simulink model "suspension2DOF"  (R2025b)
settings: Solver=ode5  StartTime=0.0  StopTime=10.0  FixedStep=0.001  RelTol=1e-3
InitFcn:
  | % 悬架参数
  | m_s = 350;
  | m_u = 45;
  | k_s = 20000;
  | c_s = 1100;
  | k_t = 200000;
undefined symbols (not defined in the file): road
settings Model: Creator=23649  LastModifiedBy=23649

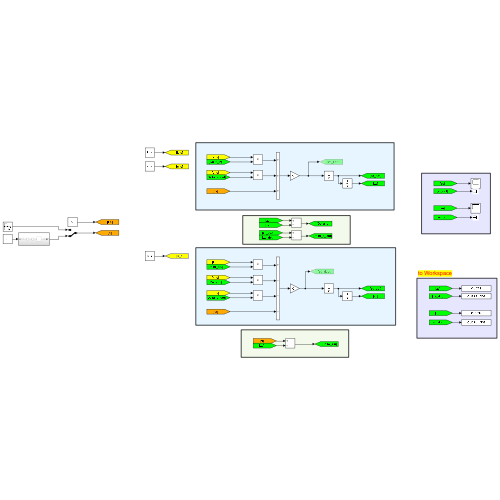
[thumbnail: Simulink's stored preview of the top-level diagram]
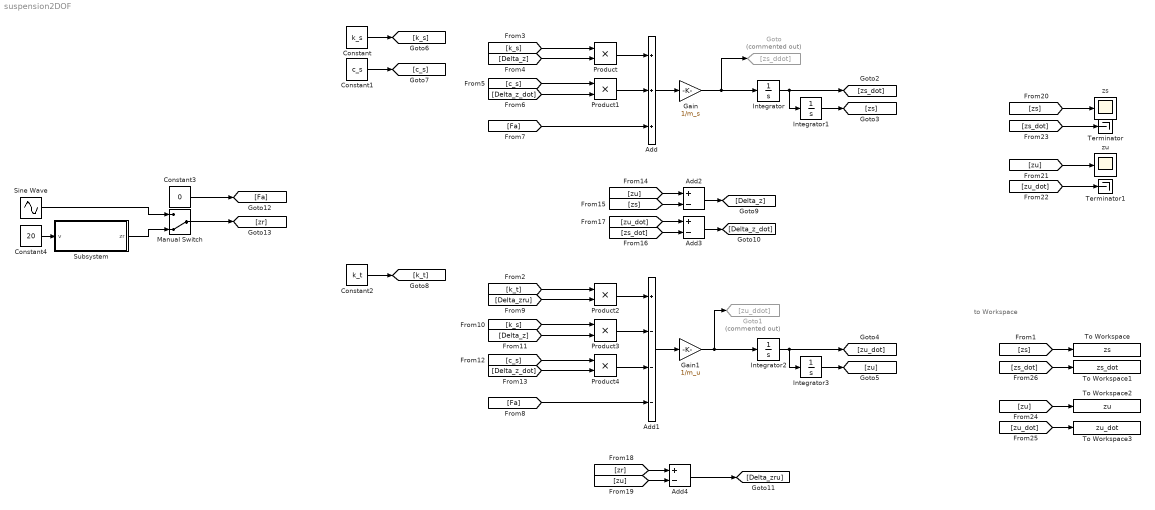
== system suspension2DOF ==
  note: to Workspace
  Add : Sum  Inputs=+++
  Add1 : Sum  Inputs=+---
  Add2 : Sum  Inputs=+-
  Add3 : Sum  Inputs=+-
  Add4 : Sum  Inputs=+-
  Constant : Constant  Value=k_s
  Constant1 : Constant  Value=c_s
  Constant2 : Constant  Value=k_t
  Constant3 : Constant  Value=0
  Constant4 : Constant  Value=20
  Gain : Gain  Gain=1/m_s
  Gain1 : Gain  Gain=1/m_u
  Goto : Goto  Commented=on  GotoTag=zs_ddot
  Goto1 : Goto  Commented=on  GotoTag=zu_ddot
  Integrator{,1..3} (4 alike) : Integrator
  Manual Switch : ManualSwitch  CurrentSetting=0
  Product{,1..4} (5 alike) : Product
  Sine Wave : Sin  Frequency=10  SampleTime=0
  Subsystem : Subsystem
  Terminator : Terminator
  Terminator1 : Terminator
  To Workspace : ToWorkspace  VariableName=zs  SampleTime=-1
  To Workspace1 : ToWorkspace  VariableName=zs_dot  SampleTime=-1
  To Workspace2 : ToWorkspace  VariableName=zu  SampleTime=-1
  To Workspace3 : ToWorkspace  VariableName=zu_dot  SampleTime=-1
  zs : Scope
      settings: ActiveDisplayYMinimum=-0.09781656463935004  ActiveDisplayYMaximum=0.084748231239210714
  zu : Scope
      settings: ActiveDisplayYMinimum=-0.097978742792255435  ActiveDisplayYMaximum=0.080113596148861266
  wires:
  Product/1 -> Add/1
  [Delta_z] -> Product/2
  [k_s] -> Product/1
  Product1/1 -> Add/2
  [Fa] -> Add/3
  [Delta_z_dot] -> Product1/2
  [c_s] -> Product1/1
  Add/1 -> Gain/1
  Gain/1 -> Goto/1, Integrator/1
  Integrator/1 -> [zs_dot], Integrator1/1
  Integrator1/1 -> [zs]
  Integrator3/1 -> [zu]
  Integrator2/1 -> Integrator3/1, [zu_dot]
  Gain1/1 -> Integrator2/1, Goto1/1
  Add1/1 -> Gain1/1
  [k_s] -> Product3/1
  [Delta_z] -> Product3/2
  Product3/1 -> Add1/2
  [k_t] -> Product2/1
  [Delta_zru] -> Product2/2
  Product2/1 -> Add1/1
  Constant/1 -> [k_s]
  Constant1/1 -> [c_s]
  Constant2/1 -> [k_t]
  [c_s] -> Product4/1
  [Delta_z_dot] -> Product4/2
  [Fa] -> Add1/4
  Product4/1 -> Add1/3
  [zu] -> Add2/1
  [zs] -> Add2/2
  Add2/1 -> [Delta_z]
  [zu_dot] -> Add3/1
  [zs_dot] -> Add3/2
  Add3/1 -> [Delta_z_dot]
  [zu] -> Add4/2
  [zr] -> Add4/1
  Add4/1 -> [Delta_zru]
  [zs] -> zs/1
  [zu] -> zu/1
  [zs_dot] -> Terminator/1
  [zu_dot] -> Terminator1/1
  Constant3/1 -> [Fa]
  Manual Switch/1 -> [zr]
  Constant4/1 -> Subsystem/1(v)
  Sine Wave/1 -> Manual Switch/1
  Subsystem/1(zr) -> Manual Switch/2
  [zs] -> To Workspace/1
  [zs_dot] -> To Workspace1/1
  [zu] -> To Workspace2/1
  [zu_dot] -> To Workspace3/1

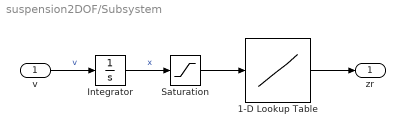
== system suspension2DOF/Subsystem ==
  v : Inport
  1-D Lookup Table : Lookup_n-D  NumberOfTableDimensions=1  BreakpointsForDimension1=road.x  Table=road.z  ExtrapMethod=Clip  InternalRulePriority=Speed  RndMeth=Simplest
  Integrator : Integrator
  Saturation : Saturate  UpperLimit=road.L-road.dx  LowerLimit=0
  zr : Outport
  wires:
  v/1 -> Integrator/1  "v"
  Integrator/1 -> Saturation/1  "x"
  Saturation/1 -> 1-D Lookup Table/1
  1-D Lookup Table/1 -> zr/1
